simulink model "realtime_test"  (R2017a)
settings: Solver=VariableStepAuto  StartTime=0.0  StopTime=inf  RelTol=1e-3
PostLoadFcn:
  | cd(fileparts(which(bdroot)))
InitFcn:
  | addpath(genpath('../'));arm_datafile
StartFcn:
  | h = bindCallback
model workspace (MAT data in the model file):
  app : r3d3 (value not decoded)
libraries: sldrtlib x1
CloseFcn:
  | hws = get_param(bdroot,'ModelWorkspace');hws.clear('app')
settings Model: Creator=Ortix  LastModifiedBy=Ortix

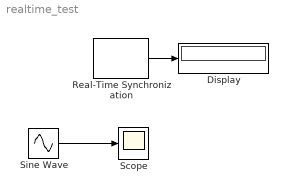
== system realtime_test ==
  Display : Display
  Real-Time Synchronization : sldrtlib/Real-Time Synchronization  SampleTime=0.1  MaxMissedTicks=100  ShowMissedTicks=on  YieldWhenWaiting=off
  Scope : Scope
  Sine Wave : Sin  SampleTime=0
  wires:
  Sine Wave/1 -> Scope/1
  Real-Time Synchronization/1 -> Display/1
